simulink model "ss_model"  (R2016b)
settings: Solver=VariableStepAuto  StartTime=0.0  StopTime=10.0  RelTol=1e-3  EnableMultiTasking=on
undefined symbols (not defined in the file): A1, A2, B1, B2, C1, C2, D1, D2
libraries: simulink_extras x2
settings Model: Creator=roslovetspv  LastModifiedBy=roslovetspv
settings OptimizationCC: LifeSpan=inf
settings DebuggingCC: SFUnexpectedBacktrackingDiag=warning  SFNoUnconditionalDefaultTransitionDiag=warning  SFExecutionAtInitializationDiag=none
settings GRTTargetCC: TargetLangStandard=C89/C90 (ANSI)  GeneratePreprocessorConditionals=Disable all
settings ConfigComp: CovMetricSettings=dw  CovHtmlReporting=on  CovSaveCumulativeToWorkspaceVar=on  CovSaveSingleToWorkspaceVar=on  CovExternalEMLEnable=off

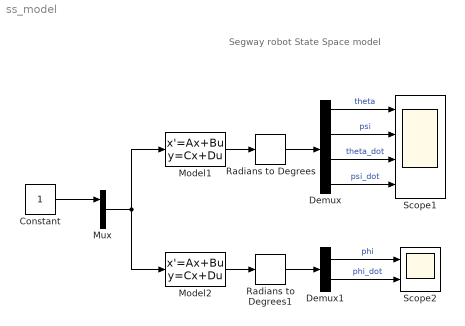
== system ss_model ==
  note: Segway robot State Space model
  Constant : Constant
  Demux : Demux
  Demux1 : Demux  Outputs=2
  Model1 : StateSpace  A=A1  B=B1  C=C1  D=D1  X0=0
  Model2 : StateSpace  A=A2  B=B2  C=C2  D=D2  X0=0
  Mux : Mux  Inputs=2
  Radians to Degrees : simulink_extras/Transformations/Radians to Degrees
  Radians to Degrees1 : simulink_extras/Transformations/Radians to Degrees
  Scope1 : Scope  NumInputPorts=4
  Scope2 : Scope  NumInputPorts=2
  wires:
  Mux/1 -> Model2/1, Model1/1
  Model1/1 -> Radians to Degrees/1
  Demux/1 -> Scope1/1  "theta"
  Demux/2 -> Scope1/2  "psi"
  Demux/3 -> Scope1/3  "theta_dot"
  Demux/4 -> Scope1/4  "psi_dot"
  Radians to Degrees/1 -> Demux/1
  Model2/1 -> Radians to Degrees1/1
  Demux1/1 -> Scope2/1  "phi"
  Demux1/2 -> Scope2/2  "phi_dot"
  Radians to Degrees1/1 -> Demux1/1
  Constant/1 -> Mux/1
